simulink model "M10B39_es_V1"  (R2024b)
settings: Solver=ode23tb  StartTime=0.0  StopTime=20  FixedStep=0.001  RelTol=1e-3  EnableMultiTasking=on
InitFcn:
  | initAll;
values from neighbouring files (symbols this model uses):
  acom = 100    [initAll_V1.m]    (also in initAll_V2.m; initAll_V3.m; parameterinit.mat)
  AVm0 = [4.26082678503 4.656135219]    [parameterinit.mat]
  bcom = 50    [initAll_V1.m]    (also in initAll_V2.m; initAll_V3.m; parameterinit.mat)
  commun = 0*commun    [initAll_V1.m]    (also in initAll_V2.m; initAll_V3.m; parameterinit.mat = [0  0  0; 0  0  0; 0  0  0; 0  0  0])
  DataDelay = 0.0*DataDelay    [initAll_V1.m]    (also in initAll_V2.m; initAll_V3.m; parameterinit.mat = [0  0  0; 0  0  0; 0  0  0; 0  0  0])
  ESinit =     [parameterinit.mat]
  fB = 50    [initAll.m]    (also in initAll_V1.m; initAll_V2.m; initAll_V3.m; parameterinit.mat)
  Geninit = Generator_init(opdata,SynMach_in_gidx)    [initAll.m]    (also in initAll_V1.m; initAll_V2.m; initAll_V3.m = Generator_init(opdata_all,SynMach_in_gidx1); parameterinit.mat = )
  lam = 100    [initAll_V1.m]    (also in initAll_V2.m; initAll_V3.m; parameterinit.mat)
  SgridB = 100    [initAll.m]    (also in initAll_V1.m; initAll_V2.m; initAll_V3.m; parameterinit.mat)
  wB = 2*pi*fB    (= 314.159265359)    [initAll.m]    (also in initAll_V1.m; initAll_V2.m; initAll_V3.m; parameterinit.mat)
  Windinit =     [parameterinit.mat]
  YY_load = [3.65450097002 -2.05705688056 0 0 0 0 0 0 0 0 0 0 ... (1521 elements, 39x39)]    [parameterinit.mat]    (also in powerflowcaculate.m = full(YY))
undefined symbols (not defined in the file or in its folder): c1, c2, c3, c4, c5, c6, cp_nom, lambda_nom, P_wind_base, Pelec_base, Pnom
libraries: spsBistableLib x12, simulink_extras x4, slpidlib x1, simulink x1
(part 2 of 7)

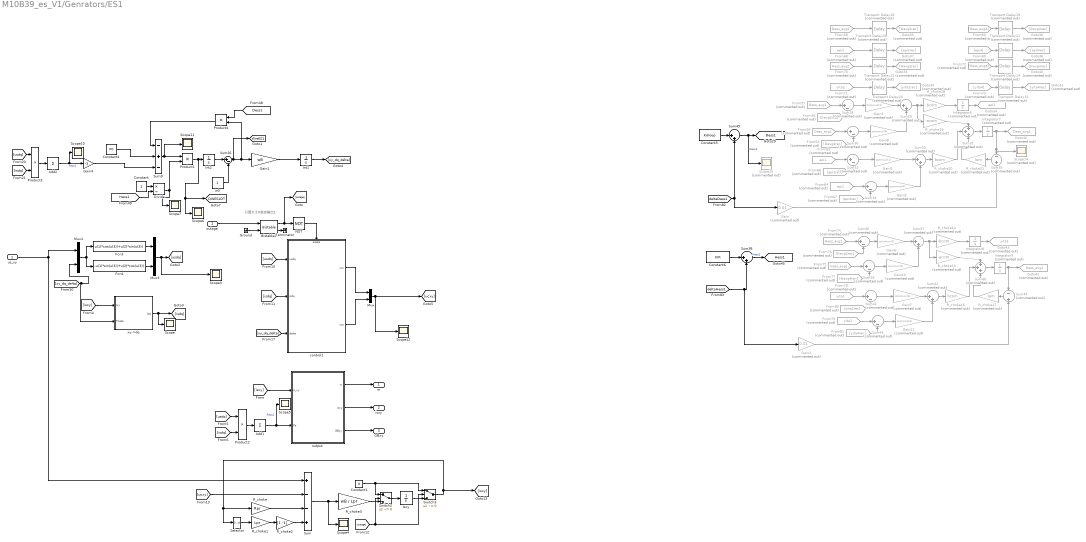
== system M10B39_es_V1/Genrators/ES1 ==
  note: 只要大于0就会输出1
  us_xy : Inport
  outage : Inport  Port=2
  " control1" : Subsystem
  Add1 : Sum  Inputs=+
  Add2 : Sum  Inputs=+
  Bistable2 : spsBistableLib/Bistable  Qpriority=Set  ic=0  Ts=0
      settings: LibrarySourceBlock=sps_lib/Control/Bistable
  Constant : Constant
  Constant1 : Constant  Value=0
  Constant4 : Constant  Value=P0
  Constant5 : Constant  Value=Kdroop
  Constant6 : Constant  Value=KIR
  Divide : Product  Inputs=*/
  Fcn3 : Fcn  Expr=u(1)*cos(u(3))+u(2)*sin(u(3))
  Fcn4 : Fcn  Expr=-u(1)*sin(u(3))+u(2)*cos(u(3))
  From57 : From  Commented=on  GotoTag=Dess_avg1  TagVisibility=global
  From58 : From  Commented=on  GotoTag=Dess_avg2  TagVisibility=global
  From59 : From  Commented=on  GotoTag=Dess_avg1  TagVisibility=global
  From60 : From  Commented=on  GotoTag=Dess_avg4  TagVisibility=global
  From61 : From  Commented=on  GotoTag=Davg2rec
  From62 : From  Commented=on  GotoTag=Davg4rec
  From63 : From  Commented=on  GotoTag=epi1  TagVisibility=global
  From64 : From  Commented=on  GotoTag=epi1  TagVisibility=global
  From66 : From  Commented=on  GotoTag=epi2rec
  From67 : From  Commented=on  GotoTag=epi4rec
  From68 : From  Commented=on  GotoTag=epi2  TagVisibility=global
  From69 : From  Commented=on  GotoTag=epi4  TagVisibility=global
  From70 : From  Commented=on  GotoTag=Hess_avg2  TagVisibility=global
  From71 : From  Commented=on  GotoTag=yita2  TagVisibility=global
  From72 : From  Commented=on  GotoTag=Hess_avg4  TagVisibility=global
  From73 : From  Commented=on  GotoTag=yita4  TagVisibility=global
  From74 : From  Commented=on  GotoTag=Hess_avg1  TagVisibility=global
  From75 : From  Commented=on  GotoTag=Hess_avg1  TagVisibility=global
  From76 : From  Commented=on  GotoTag=Havg2rec
  From77 : From  Commented=on  GotoTag=Havg4rec
  From78 : From  Commented=on  GotoTag=yita1  TagVisibility=global
  From79 : From  Commented=on  GotoTag=yita1  TagVisibility=global
  From80 : From  Commented=on  GotoTag=yita2rec
  From81 : From  Commented=on  GotoTag=yita4rec
  Gain : Gain  Commented=on  Gain=0.01
  Gain1 : Gain  Gain=wB  SaturateOnIntegerOverflow=on  OutDataTypeStr=Inherit: Same as input  ParamDataTypeStr=Inherit: Same as input
  Gain{8..11} (4 alike) : Gain  Commented=on  Gain=commun(4)
  Gain2 : Gain  Commented=on  Gain=0.01
  Gain{3,5..7} (4 alike) : Gain  Commented=on  Gain=commun(1)
  Gain4 : Gain  Gain=-1
  Goto32 : Goto  Commented=on  GotoTag=Dess_avg1  TagVisibility=global
  Goto33 : Goto  Commented=on  GotoTag=Havg2rec
  Goto34 : Goto  Commented=on  GotoTag=epi1  TagVisibility=global
  Goto35 : Goto  Commented=on  GotoTag=Davg2rec
  Goto36 : Goto  Commented=on  GotoTag=Davg4rec
  Goto37 : Goto  Commented=on  GotoTag=epi2rec
  Goto38 : Goto  Commented=on  GotoTag=epi4rec
  Goto39 : Goto  Commented=on  GotoTag=yita2rec
  Goto40 : Goto  Commented=on  GotoTag=Havg4rec
  Goto41 : Goto  Commented=on  GotoTag=yita4rec
  Goto42 : Goto  Commented=on  GotoTag=Hess_avg1  TagVisibility=global
  Goto43 : Goto  Commented=on  GotoTag=yita1  TagVisibility=global
  Ground : Ground
  Int1 : Integrator  InitialCondition=Dels_hvdc
  Int2 : Integrator  InitialCondition=1
  Integrator{6..9} (4 alike) : Integrator  Commented=on
  Isxy : Integrator  InitialCondition=[Is_xA_0 Is_yA_0]
  Mux : Mux  Inputs=2
  Mux3 : Mux  Inputs=2
  Mux4 : Mux  Inputs=2
  NOT : Logic  Operator=NOT  AllPortsSameDT=off  OutDataTypeStr=boolean
  Product1 : Product
  Product2 : Product  RndMeth=Zero
  Product3 : Product  RndMeth=Zero
  Product4 : Product
  R_choke : Gain  Gain=Rpr  SaturateOnIntegerOverflow=on  OutDataTypeStr=Inherit: Same as input  ParamDataTypeStr=Inherit: Same as input
  R_choke1 : Gain  Gain=Lpr  SaturateOnIntegerOverflow=on  OutDataTypeStr=Inherit: Same as input  ParamDataTypeStr=Inherit: Same as input
  R_choke14 : Gain  Commented=on  Gain=-bcom  SaturateOnIntegerOverflow=on  OutDataTypeStr=Inherit: Same as input  ParamDataTypeStr=Inherit: Same as input
  R_choke15 : Gain  Commented=on  Gain=-acom  SaturateOnIntegerOverflow=on  OutDataTypeStr=Inherit: Same as input  ParamDataTypeStr=Inherit: Same as input
  R_choke16 : Gain  Commented=on  Gain=bcom  SaturateOnIntegerOverflow=on  OutDataTypeStr=Inherit: Same as input  ParamDataTypeStr=Inherit: Same as input
  R_choke17 : Gain  Commented=on  Gain=lam  SaturateOnIntegerOverflow=on  OutDataTypeStr=Inherit: Same as input  ParamDataTypeStr=Inherit: Same as input
  R_choke18 : Gain  Commented=on  Gain=-bcom  SaturateOnIntegerOverflow=on  OutDataTypeStr=Inherit: Same as input  ParamDataTypeStr=Inherit: Same as input
  R_choke19 : Gain  Commented=on  Gain=-acom  SaturateOnIntegerOverflow=on  OutDataTypeStr=Inherit: Same as input  ParamDataTypeStr=Inherit: Same as input
  R_choke2 : Gain  Gain=[1 -1]  SaturateOnIntegerOverflow=on  OutDataTypeStr=Inherit: Same as input  ParamDataTypeStr=Inherit: Same as input
  R_choke20 : Gain  Commented=on  Gain=bcom  SaturateOnIntegerOverflow=on  OutDataTypeStr=Inherit: Same as input  ParamDataTypeStr=Inherit: Same as input
  R_choke21 : Gain  Commented=on  Gain=lam  SaturateOnIntegerOverflow=on  OutDataTypeStr=Inherit: Same as input  ParamDataTypeStr=Inherit: Same as input
  R_choke3 : Gain  Gain=wB / Lpr  SaturateOnIntegerOverflow=on  OutDataTypeStr=Inherit: Same as input  ParamDataTypeStr=Inherit: Same as input
  Scope{,3..7,10..12} (9 alike) : Scope
  Scope14 : Scope  Commented=on
  Scope15 : Scope  Commented=on
  Selector : Selector  InputPortWidth=2  IndexOptions=Index vector (dialog)  Indices=[2 1]  OutputSizes=1
  Sum : Sum  Inputs=+--+  SaturateOnIntegerOverflow=on
  Sum26 : Sum  Inputs=|+-  SaturateOnIntegerOverflow=on
  Sum{28,30,32,34,36,39,41,43} (8 alike) : Sum  Commented=on  Inputs=|+-  SaturateOnIntegerOverflow=on
  Sum{29,33,37,42} (4 alike) : Sum  Commented=on  Inputs=|++  SaturateOnIntegerOverflow=on
  Sum31 : Sum  Commented=on  Inputs=+++  SaturateOnIntegerOverflow=on
  Sum35 : Sum  Commented=on  Inputs=-+  SaturateOnIntegerOverflow=on
  Sum38 : Sum  Inputs=|++  SaturateOnIntegerOverflow=on
  Sum40 : Sum  Commented=on  Inputs=+++  SaturateOnIntegerOverflow=on
  Sum44 : Sum  Commented=on  Inputs=-+  SaturateOnIntegerOverflow=on
  Sum45 : Sum  Inputs=|++  SaturateOnIntegerOverflow=on
  Sum9 : Sum  Inputs=-+-  SaturateOnIntegerOverflow=on
  Switch2 : Switch  Criteria=u2 ~= 0  Threshold=0.5  InputSameDT=off
  Switch3 : Switch  Criteria=u2 ~= 0  Threshold=0.5  InputSameDT=off
  Terminator : Terminator
  Transport Delay{14..15,19,21} (4 alike) : TransportDelay  Commented=on  DelayTime=DataDelay(4,2)
  Transport Delay{18,20,22..23} (4 alike) : TransportDelay  Commented=on  DelayTime=DataDelay(2,1)
  output : Subsystem
  w0 : Constant
  xy->dq : Subsystem
  m : Outport
  isxy : Outport  Port=2
  GBxy : Outport  Port=3
  tag scope: DWES1DT=global, Dess1=global, Hess1=global, WreES1=global
  wires:
  Selector/1 -> R_choke1/1
  Sum/1 -> Scope4/1, R_choke3/1
  R_choke3/1 -> Switch2/3
  Ground/1 -> Bistable2/2
  R_choke2/1 -> Sum/4
  R_choke/1 -> Sum/3
  [ucxy] -> Sum/2
  output/1(m) -> m/1
  NOT/1 -> " control1"/Enable
  R_choke1/1 -> R_choke2/1
  Bistable2/1 -> NOT/1, [outage]
  Isxy/1 -> Switch3/3
  [isxy] -> xy->dq/1(Ixy)
  [isxy] -> output/1(is_xy)
  output/2(isxy) -> isxy/1
  [xy_dq_delta] -> " control1"/3(delta)
  xy->dq/1(Idq) -> [isdq], Scope/1
  Bistable2/2 -> Terminator/1
  outage/1 -> Bistable2/1
  [outage] -> Switch2/2, Switch3/2
  [isdq] -> " control1"/2(isdq)
  " control1"/1(ucx) -> Mux/1
  Switch2/1 -> Isxy/1
  Switch3/1 -> R_choke/1, Selector/1, [isxy]
  Mux/1 -> Scope12/1, [ucxy]
  [usdq] -> " control1"/1(usdq)
  output/3(GBxy) -> GBxy/1
  Constant1/1 -> Switch2/1, Switch3/1
  " control1"/2(ucy) -> Mux/2
  [usdq] -> Product2/1
  Add1/1 -> Scope5/1, output/2(Pe)  "Pess1"
  Product2/1 -> Add1/1
  [isdq] -> Product2/2
  Product1/1 -> Scope6/1, [DWES1DT], Int2/1
  Sum26/1 -> [WreES1], Product4/2, Gain1/1
  Int2/1 -> Sum26/1
  w0/1 -> Sum26/2
  Sum9/1 -> Product1/1, Scope11/1
  Constant/1 -> Divide/1
  Divide/1 -> Product1/2, Scope7/1
  [Hess1] -> Divide/2
  us_xy/1 -> Mux4/1, Sum/1
  Fcn3/1 -> Mux3/1
  Fcn4/1 -> Mux3/2
  Mux4/1 -> Fcn3/1, Fcn4/1
  [xy_dq_delta] -> Mux4/2, xy->dq/2(Theta)
  Mux3/1 -> Scope3/1, [usdq]
  Gain4/1 -> Sum9/3
  Constant4/1 -> Sum9/2
  Product4/1 -> Sum9/1
  Int1/1 -> [xy_dq_delta]
  Add2/1 -> Gain4/1, Scope10/1  "Pess1"
  [usdq] -> Product3/1
  [isdq] -> Product3/2
  Product3/1 -> Add2/1
  Transport Delay19/1 -> Goto36/1
  R_choke20/1 -> Sum31/2
  R_choke19/1 -> Sum31/1
  From57/1 -> Sum28/1
  From59/1 -> Sum30/1
  Sum38/1 -> [Hess1]  "Hess1"
  Sum45/1 -> Scope15/1, [Dess1]  "Dess1"
  Constant6/1 -> Sum38/1
  From64/1 -> Sum34/1
  R_choke21/1 -> Sum31/3
  Integrator6/1 -> Goto34/1
  Sum35/1 -> R_choke21/1
  Sum31/1 -> Integrator7/1
  Integrator7/1 -> Goto32/1, Scope14/1, Sum35/1
  Transport Delay21/1 -> Goto38/1
  From68/1 -> Transport Delay20/1
  From67/1 -> Sum34/2
  From62/1 -> Sum30/2
  From80/1 -> Sum41/2
  From78/1 -> Sum41/1
  Sum40/1 -> Integrator9/1
  [deltaDess1] -> Sum45/2, Gain/1
  R_choke18/1 -> Integrator6/1
  From77/1 -> Sum39/2
  From63/1 -> Sum32/1
  From76/1 -> Sum36/2
  Sum42/1 -> R_choke16/1
  From58/1 -> Transport Delay18/1
  Transport Delay20/1 -> Goto37/1
  Transport Delay14/1 -> Goto40/1
  From75/1 -> Sum39/1
  Integrator9/1 -> Goto42/1, Sum44/1
  Sum29/1 -> R_choke19/1, R_choke18/1
  From61/1 -> Sum28/2
  From71/1 -> Transport Delay23/1
  Sum37/1 -> R_choke15/1, R_choke14/1
  R_choke14/1 -> Integrator8/1
  Integrator8/1 -> Goto43/1
  Transport Delay18/1 -> Goto35/1
  R_choke17/1 -> Sum40/3
  R_choke15/1 -> Sum40/1
  R_choke16/1 -> Sum40/2
  From74/1 -> Sum36/1
  [deltaHess1] -> Sum38/2, Gain2/1
  Sum44/1 -> R_choke17/1
  Sum33/1 -> R_choke20/1
  Transport Delay23/1 -> Goto39/1
  From66/1 -> Sum32/2
  Transport Delay22/1 -> Goto33/1
  Transport Delay15/1 -> Goto41/1
  From70/1 -> Transport Delay22/1
  [Dess1] -> Product4/1
  Gain1/1 -> Int1/1
  From81/1 -> Sum43/2
  From79/1 -> Sum43/1
  Gain/1 -> Sum35/2
  Gain2/1 -> Sum44/2
  From60/1 -> Transport Delay19/1
  From69/1 -> Transport Delay21/1
  From72/1 -> Transport Delay14/1
  From73/1 -> Transport Delay15/1
  Gain3/1 -> Sum29/1
  Sum28/1 -> Gain3/1
  Gain5/1 -> Sum33/1
  Sum32/1 -> Gain5/1
  Sum36/1 -> Gain6/1
  Gain6/1 -> Sum37/1
  Gain7/1 -> Sum42/1
  Sum41/1 -> Gain7/1
  Sum30/1 -> Gain8/1
  Gain8/1 -> Sum29/2
  Sum34/1 -> Gain9/1
  Gain9/1 -> Sum33/2
  Sum39/1 -> Gain10/1
  Gain10/1 -> Sum37/2
  Sum43/1 -> Gain11/1
  Gain11/1 -> Sum42/2
  Constant5/1 -> Sum45/1

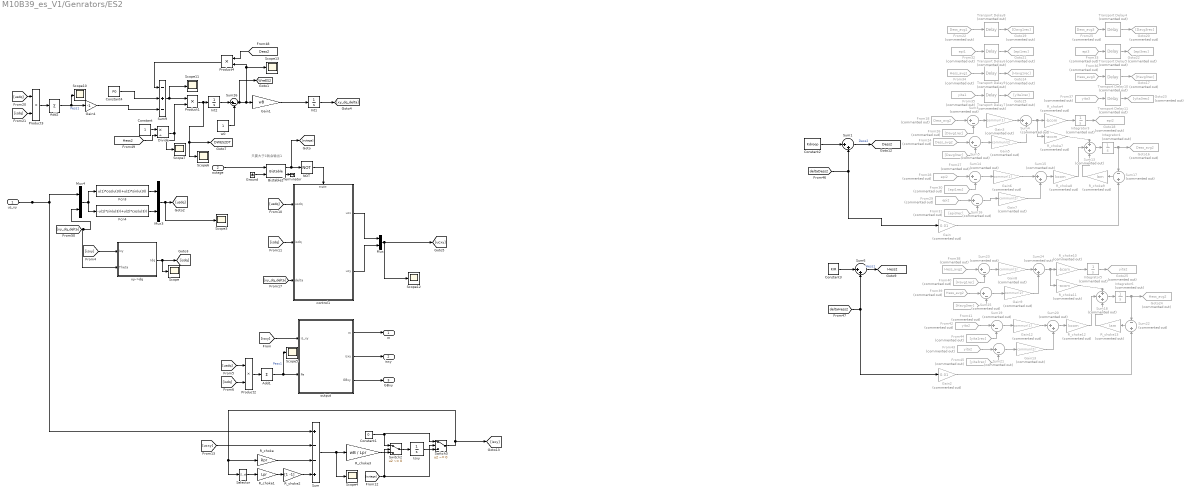
== system M10B39_es_V1/Genrators/ES2 ==
  note: 只要大于0就会输出1
  us_xy : Inport
  outage : Inport  Port=2
  " control1" : Subsystem
  Add1 : Sum  Inputs=+
  Add2 : Sum  Inputs=+
  Bistable2 : spsBistableLib/Bistable  Qpriority=Set  ic=0  Ts=0
      settings: LibrarySourceBlock=sps_lib/Control/Bistable
  Constant : Constant
  Constant1 : Constant  Value=0
  Constant2 : Constant  Value=Kdroop
  Constant3 : Constant  Value=KIR
  Constant4 : Constant  Value=P0
  Divide : Product  Inputs=*/
  Fcn3 : Fcn  Expr=u(1)*cos(u(3))+u(2)*sin(u(3))
  Fcn4 : Fcn  Expr=-u(1)*sin(u(3))+u(2)*cos(u(3))
  From18 : From  Commented=on  GotoTag=Dess_avg2  TagVisibility=global
  From22 : From  Commented=on  GotoTag=Dess_avg1  TagVisibility=global
  From24 : From  Commented=on  GotoTag=Dess_avg2  TagVisibility=global
  From25 : From  Commented=on  GotoTag=Dess_avg3  TagVisibility=global
  From26 : From  Commented=on  GotoTag=Davg1rec
  From27 : From  Commented=on  GotoTag=Davg3rec
  From28 : From  Commented=on  GotoTag=epi2  TagVisibility=global
  From29 : From  Commented=on  GotoTag=epi2  TagVisibility=global
  From30 : From  Commented=on  GotoTag=epi1rec
  From31 : From  Commented=on  GotoTag=epi3rec
  From32 : From  Commented=on  GotoTag=epi1  TagVisibility=global
  From33 : From  Commented=on  GotoTag=epi3  TagVisibility=global
  From34 : From  Commented=on  GotoTag=Hess_avg1  TagVisibility=global
  From35 : From  Commented=on  GotoTag=yita1  TagVisibility=global
  From36 : From  Commented=on  GotoTag=Hess_avg3  TagVisibility=global
  From37 : From  Commented=on  GotoTag=yita3  TagVisibility=global
  From38 : From  Commented=on  GotoTag=Hess_avg2  TagVisibility=global
  From39 : From  Commented=on  GotoTag=Hess_avg2  TagVisibility=global
  From40 : From  Commented=on  GotoTag=Havg1rec
  From41 : From  Commented=on  GotoTag=Havg3rec
  From42 : From  Commented=on  GotoTag=yita2  TagVisibility=global
  From43 : From  Commented=on  GotoTag=yita2  TagVisibility=global
  From44 : From  Commented=on  GotoTag=yita1rec
  From45 : From  Commented=on  GotoTag=yita3rec
  Gain : Gain  Commented=on  Gain=0.01
  Gain1 : Gain  Gain=wB  SaturateOnIntegerOverflow=on  OutDataTypeStr=Inherit: Same as input  ParamDataTypeStr=Inherit: Same as input
  Gain{3,6,8,12} (4 alike) : Gain  Commented=on  Gain=commun(1)
  Gain{5,7,9,13} (4 alike) : Gain  Commented=on  Gain=commun(2)
  Gain2 : Gain  Commented=on  Gain=0.01
  Gain4 : Gain  Gain=-1
  Goto14 : Goto  Commented=on  GotoTag=Havg1rec
  Goto15 : Goto  Commented=on  GotoTag=yita1rec
  Goto16 : Goto  Commented=on  GotoTag=Dess_avg2  TagVisibility=global
  Goto17 : Goto  Commented=on  GotoTag=Havg3rec
  Goto18 : Goto  Commented=on  GotoTag=epi2  TagVisibility=global
  Goto19 : Goto  Commented=on  GotoTag=Davg1rec
  Goto20 : Goto  Commented=on  GotoTag=Davg3rec
  Goto21 : Goto  Commented=on  GotoTag=epi1rec
  Goto22 : Goto  Commented=on  GotoTag=epi3rec
  Goto23 : Goto  Commented=on  GotoTag=yita3rec
  Goto24 : Goto  Commented=on  GotoTag=Hess_avg2  TagVisibility=global
  Goto25 : Goto  Commented=on  GotoTag=yita2  TagVisibility=global
  Ground : Ground
  Int1 : Integrator  InitialCondition=Dels_hvdc
  Int2 : Integrator  InitialCondition=1
  Integrator{3..6} (4 alike) : Integrator  Commented=on
  Isxy : Integrator  InitialCondition=[Is_xA_0 Is_yA_0]
  Mux : Mux  Inputs=2
  Mux3 : Mux  Inputs=2
  Mux4 : Mux  Inputs=2
  NOT : Logic  Operator=NOT  AllPortsSameDT=off  OutDataTypeStr=boolean
  Product1 : Product
  Product2 : Product  RndMeth=Zero
  Product3 : Product  RndMeth=Zero
  Product4 : Product
  R_choke : Gain  Gain=Rpr  SaturateOnIntegerOverflow=on  OutDataTypeStr=Inherit: Same as input  ParamDataTypeStr=Inherit: Same as input
  R_choke1 : Gain  Gain=Lpr  SaturateOnIntegerOverflow=on  OutDataTypeStr=Inherit: Same as input  ParamDataTypeStr=Inherit: Same as input
  R_choke10 : Gain  Commented=on  Gain=-bcom  SaturateOnIntegerOverflow=on  OutDataTypeStr=Inherit: Same as input  ParamDataTypeStr=Inherit: Same as input
  R_choke11 : Gain  Commented=on  Gain=-acom  SaturateOnIntegerOverflow=on  OutDataTypeStr=Inherit: Same as input  ParamDataTypeStr=Inherit: Same as input
  R_choke12 : Gain  Commented=on  Gain=bcom  SaturateOnIntegerOverflow=on  OutDataTypeStr=Inherit: Same as input  ParamDataTypeStr=Inherit: Same as input
  R_choke13 : Gain  Commented=on  Gain=lam  SaturateOnIntegerOverflow=on  OutDataTypeStr=Inherit: Same as input  ParamDataTypeStr=Inherit: Same as input
  R_choke2 : Gain  Gain=[1 -1]  SaturateOnIntegerOverflow=on  OutDataTypeStr=Inherit: Same as input  ParamDataTypeStr=Inherit: Same as input
  R_choke3 : Gain  Gain=wB / Lpr  SaturateOnIntegerOverflow=on  OutDataTypeStr=Inherit: Same as input  ParamDataTypeStr=Inherit: Same as input
  R_choke4 : Gain  Commented=on  Gain=-bcom  SaturateOnIntegerOverflow=on  OutDataTypeStr=Inherit: Same as input  ParamDataTypeStr=Inherit: Same as input
  R_choke7 : Gain  Commented=on  Gain=-acom  SaturateOnIntegerOverflow=on  OutDataTypeStr=Inherit: Same as input  ParamDataTypeStr=Inherit: Same as input
  R_choke8 : Gain  Commented=on  Gain=bcom  SaturateOnIntegerOverflow=on  OutDataTypeStr=Inherit: Same as input  ParamDataTypeStr=Inherit: Same as input
  R_choke9 : Gain  Commented=on  Gain=lam  SaturateOnIntegerOverflow=on  OutDataTypeStr=Inherit: Same as input  ParamDataTypeStr=Inherit: Same as input
  Scope{,3..7,10..13} (10 alike) : Scope
  Selector : Selector  InputPortWidth=2  IndexOptions=Index vector (dialog)  Indices=[2 1]  OutputSizes=1
  Sum : Sum  Inputs=+--+  SaturateOnIntegerOverflow=on
  Sum1 : Sum  Inputs=|++  SaturateOnIntegerOverflow=on
  Sum13 : Sum  Commented=on  Inputs=+++  SaturateOnIntegerOverflow=on
  Sum{3,5,14,16,19,21,23,25} (8 alike) : Sum  Commented=on  Inputs=|+-  SaturateOnIntegerOverflow=on
  Sum{4,15,20,24} (4 alike) : Sum  Commented=on  Inputs=|++  SaturateOnIntegerOverflow=on
  Sum17 : Sum  Commented=on  Inputs=-+  SaturateOnIntegerOverflow=on
  Sum18 : Sum  Commented=on  Inputs=+++  SaturateOnIntegerOverflow=on
  Sum22 : Sum  Commented=on  Inputs=-+  SaturateOnIntegerOverflow=on
  Sum26 : Sum  Inputs=|+-  SaturateOnIntegerOverflow=on
  Sum6 : Sum  Inputs=|++  SaturateOnIntegerOverflow=on
  Sum9 : Sum  Inputs=-+-  SaturateOnIntegerOverflow=on
  Switch2 : Switch  Criteria=u2 ~= 0  Threshold=0.5  InputSameDT=off
  Switch3 : Switch  Criteria=u2 ~= 0  Threshold=0.5  InputSameDT=off
  Terminator : Terminator
  Transport Delay{4..5,10..11} (4 alike) : TransportDelay  Commented=on  DelayTime=DataDelay(3,1)
  Transport Delay{6..9} (4 alike) : TransportDelay  Commented=on  DelayTime=DataDelay(1,2)
  output : Subsystem
  w0 : Constant
  xy->dq : Subsystem
  m : Outport
  isxy : Outport  Port=2
  GBxy : Outport  Port=3
  tag scope: DWES2DT=global, Dess2=global, Hess2=global, WreES2=global
  wires:
  Selector/1 -> R_choke1/1
  Sum/1 -> Scope4/1, R_choke3/1
  R_choke3/1 -> Switch2/3
  Ground/1 -> Bistable2/2
  R_choke2/1 -> Sum/4
  R_choke/1 -> Sum/3
  [ucxy] -> Sum/2
  output/1(m) -> m/1
  NOT/1 -> " control1"/Enable
  R_choke1/1 -> R_choke2/1
  Bistable2/1 -> NOT/1, [outage]
  Isxy/1 -> Switch3/3
  [isxy] -> xy->dq/1(Ixy)
  [isxy] -> output/1(is_xy)
  output/2(isxy) -> isxy/1
  [xy_dq_delta] -> " control1"/3(delta)
  xy->dq/1(Idq) -> [isdq], Scope/1
  Bistable2/2 -> Terminator/1
  outage/1 -> Bistable2/1
  [outage] -> Switch2/2, Switch3/2
  [isdq] -> " control1"/2(isdq)
  " control1"/1(ucx) -> Mux/1
  Switch2/1 -> Isxy/1
  Switch3/1 -> R_choke/1, Selector/1, [isxy]
  Mux/1 -> Scope12/1, [ucxy]
  [usdq] -> " control1"/1(usdq)
  output/3(GBxy) -> GBxy/1
  Constant1/1 -> Switch2/1, Switch3/1
  " control1"/2(ucy) -> Mux/2
  [usdq] -> Product2/1
  Add1/1 -> output/2(Pe), Scope5/1  "Pess1"
  Product2/1 -> Add1/1
  [isdq] -> Product2/2
  Product1/1 -> Scope6/1, [DWES2DT], Int2/1
  Sum26/1 -> [WreES2], Scope13/1, Product4/2, Gain1/1
  Int2/1 -> Sum26/1
  w0/1 -> Sum26/2
  Sum9/1 -> Product1/1, Scope11/1
  Constant/1 -> Divide/1
  Divide/1 -> Product1/2, Scope7/1
  [Hess2] -> Divide/2
  us_xy/1 -> Mux4/1, Sum/1
  Fcn3/1 -> Mux3/1
  Fcn4/1 -> Mux3/2
  Mux4/1 -> Fcn3/1, Fcn4/1
  [xy_dq_delta] -> Mux4/2, xy->dq/2(Theta)
  Mux3/1 -> Scope3/1, [usdq]
  Gain4/1 -> Sum9/3
  Constant4/1 -> Sum9/2
  Product4/1 -> Sum9/1
  Int1/1 -> [xy_dq_delta]
  Add2/1 -> Gain4/1, Scope10/1  "Pess1"
  [usdq] -> Product3/1
  [isdq] -> Product3/2
  Product3/1 -> Add2/1
  [Dess2] -> Product4/1
  Gain1/1 -> Int1/1
  From27/1 -> Sum5/2
  R_choke7/1 -> Sum13/1
  From44/1 -> Sum19/2
  R_choke8/1 -> Sum13/2
  From24/1 -> Sum5/1
  From18/1 -> Sum3/1
  Transport Delay9/1 -> Goto14/1
  From26/1 -> Sum3/2
  Transport Delay6/1 -> Goto21/1
  Integrator3/1 -> Goto18/1
  From30/1 -> Sum14/2
  Transport Delay5/1 -> Goto22/1
  Sum20/1 -> R_choke12/1
  Transport Delay4/1 -> Goto20/1
  From43/1 -> Sum21/1
  Transport Delay7/1 -> Goto15/1
  Sum17/1 -> R_choke9/1
  [deltaDess2] -> Sum1/2, Gain/1
  From39/1 -> Sum25/1
  Sum13/1 -> Integrator4/1
  R_choke10/1 -> Integrator5/1
  Sum15/1 -> R_choke8/1
  R_choke9/1 -> Sum13/3
  Constant3/1 -> Sum6/1
  Integrator4/1 -> Goto16/1, Sum17/1
  From29/1 -> Sum16/1
  [deltaHess2] -> Sum6/2, Gain2/1
  Transport Delay10/1 -> Goto17/1
  From31/1 -> Sum16/2
  Sum24/1 -> R_choke11/1, R_choke10/1
  Sum6/1 -> [Hess2]  "Hess1"
  From42/1 -> Sum19/1
  From28/1 -> Sum14/1
  R_choke12/1 -> Sum18/2
  From38/1 -> Sum23/1
  R_choke11/1 -> Sum18/1
  R_choke4/1 -> Integrator3/1
  Sum4/1 -> R_choke7/1, R_choke4/1
  From45/1 -> Sum21/2
  From40/1 -> Sum23/2
  From41/1 -> Sum25/2
  Transport Delay11/1 -> Goto23/1
  Sum22/1 -> R_choke13/1
  Integrator6/1 -> Goto24/1, Sum22/1
  Sum18/1 -> Integrator6/1
  Integrator5/1 -> Goto25/1
  R_choke13/1 -> Sum18/3
  Transport Delay8/1 -> Goto19/1
  Sum1/1 -> [Dess2]  "Dess2"
  Constant2/1 -> Sum1/1
  Gain/1 -> Sum17/2
  Gain2/1 -> Sum22/2
  From22/1 -> Transport Delay8/1
  From32/1 -> Transport Delay6/1
  From34/1 -> Transport Delay9/1
  From35/1 -> Transport Delay7/1
  From25/1 -> Transport Delay4/1
  From33/1 -> Transport Delay5/1
  From36/1 -> Transport Delay10/1
  From37/1 -> Transport Delay11/1
  Gain3/1 -> Sum4/1
  Sum3/1 -> Gain3/1
  Sum5/1 -> Gain5/1
  Gain5/1 -> Sum4/2
  Gain6/1 -> Sum15/1
  Sum14/1 -> Gain6/1
  Sum16/1 -> Gain7/1
  Gain7/1 -> Sum15/2
  Sum23/1 -> Gain8/1
  Gain8/1 -> Sum24/1
  Sum25/1 -> Gain9/1
  Gain9/1 -> Sum24/2
  Gain12/1 -> Sum20/1
  Sum19/1 -> Gain12/1
  Sum21/1 -> Gain13/1
  Gain13/1 -> Sum20/2

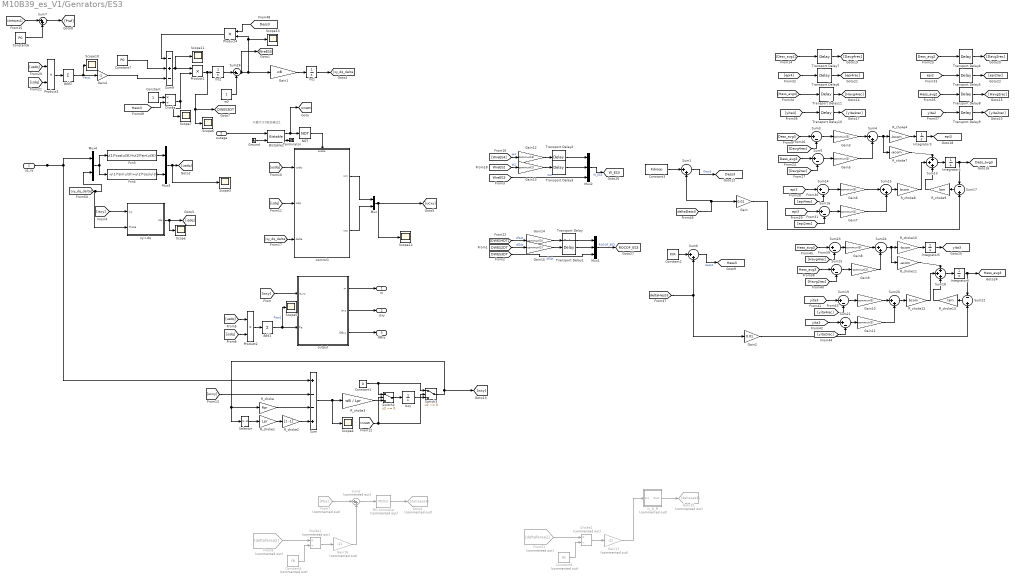
== system M10B39_es_V1/Genrators/ES3 ==
  note: 只要大于0就会输出1
  us_xy : Inport
  outage : Inport  Port=2
  " control1" : Subsystem
  Add1 : Sum  Inputs=+
  Add2 : Sum  Inputs=+
  Bistable2 : spsBistableLib/Bistable  Qpriority=Set  ic=0  Ts=0
  Constant : Constant
  Constant1 : Constant  Value=0
  Constant2 : Constant  Value=KIR
  Constant3 : Constant  Value=Kdroop
  Constant4 : Constant  Commented=on  Value=fB
  Constant5 : Constant  Commented=on  Value=fB
  Constant6 : Constant  Value=P0
  Constant7 : Constant  Value=P0
  Divide : Product  Inputs=*/
  Divide1 : Product  Commented=on  Inputs=*/
  Divide2 : Product  Commented=on  Inputs=*/
  Fcn3 : Fcn  Expr=u(1)*cos(u(3))+u(2)*sin(u(3))
  Fcn4 : Fcn  Expr=-u(1)*sin(u(3))+u(2)*cos(u(3))
  From51 : From  Commented=on  GotoTag=deltafarea2  TagVisibility=global
  From7 : From  Commented=on  GotoTag=Ptie  TagVisibility=global
  From8 : From  Commented=on  GotoTag=deltafarea2  TagVisibility=global
  Gain : Gain  Gain=0.01
  Gain1 : Gain  Gain=wB  SaturateOnIntegerOverflow=on  OutDataTypeStr=Inherit: Same as input  ParamDataTypeStr=Inherit: Same as input
  Gain{3,6,8,10,12,14} (6 alike) : Gain  Gain=commun(3)
  Gain{5,7,9,11,13,15} (6 alike) : Gain  Gain=commun(2)
  Gain16 : Gain  Commented=on  Gain=-21
  Gain17 : Gain  Commented=on  Gain=-21
  Gain2 : Gain  Gain=0.01
  Gain4 : Gain  Gain=-1
  Goto10 : Goto  Commented=on  GotoTag=deltapes3
  Goto6 : Goto  Commented=on  GotoTag=deltapes3
  Ground : Ground
  Int1 : Integrator  InitialCondition=Dels_hvdc
  Int2 : Integrator  InitialCondition=1
  Integrator{3..6} (4 alike) : Integrator
  Isxy : Integrator  InitialCondition=[Is_xA_0 Is_yA_0]
  Mux : Mux  Inputs=2
  Mux1 : Mux  Inputs=3
  Mux2 : Mux  Inputs=3
  Mux3 : Mux  Inputs=2
  Mux4 : Mux  Inputs=2
  NOT : Logic  Operator=NOT  AllPortsSameDT=off  OutDataTypeStr=boolean
  PID Controller : slpidlib/PID Controller  Commented=on  Controller=PID  Form=Parallel  TimeDomain=Continuous-time  UseExternalTs=off  SampleTime=-1  IntegratorMethod=Forward Euler  FilterMethod=Forward Euler  ControllerParametersSource=internal  P=1  I=1  UseKiTs=off  D=0  UseExternalDerivativeSource=off  N=100  UseFilter=on  TunerSelectOption=Transfer Function Based (PID Tuner App)  InitialConditionSource=internal  InitialConditionForIntegrator=0  InitialConditionForFilter=0  DifferentiatorICPrevScaledInput=0  ExternalReset=none  TrackingMode=off  Kt=1  LimitOutput=off  SatLimitsSource=internal  UpperSaturationLimit=inf  LowerSaturationLimit=-inf  LinearizeAsGain=on  AntiWindupMode=none  Kb=1  LimitIntegrator=off  UpperIntegratorSaturationLimit=inf  LowerIntegratorSaturationLimit=-inf  POutMin=[]  POutMax=[]  IOutMin=[]  IOutMax=[]  DOutMin=[]  DOutMax=[]  NOutMin=[]  NOutMax=[]  SumOutMin=[]  SumOutMax=[]  SaturationOutMin=[]  SaturationOutMax=[]  PParamMin=[]  PParamMax=[]  IParamMin=[]  IParamMax=[]  DParamMin=[]  DParamMax=[]  NParamMin=[]  NParamMax=[]  KbParamMin=[]  KbParamMax=[]  KtParamMin=[]  KtParamMax=[]  KbOutMin=[]  KbOutMax=[]  KtOutMin=[]  KtOutMax=[]  IntegratorOutMin=[]  IntegratorOutMax=[]  FilterOutMin=[]  FilterOutMax=[]  SumI1OutMin=[]  SumI1OutMax=[]  SumI2OutMin=[]  SumI2OutMax=[]  SumI3OutMin=[]  SumI3OutMax=[]  SumI4OutMin=[]  SumI4OutMax=[]  SumDOutMin=[]  SumDOutMax=[]  DifferentiatorOutMin=[]  DifferentiatorOutMax=[]  FilterDiffOutCoefMin=[]  FilterDiffOutCoefMax=[]  ReciprocalOutMin=[]  ReciprocalOutMax=[]  SumDenOutMin=[]  SumDenOutMax=[]  SumNumOutMin=[]  SumNumOutMax=[]  DivideOutMin=[]  DivideOutMax=[]  UdiffTsProdOutMin=[]  UdiffTsProdOutMax=[]  NTsProdOutMin=[]  NTsProdOutMax=[]  UintegralTsProdOutMin=[]  UintegralTsProdOutMax=[]  UngainTsProdOutMin=[]  UngainTsProdOutMax=[]  ClampingZeroOutDataTypeStr=Inherit: Inherit via back propagation  ClampingZeroOutMin=[]  ClampingZeroOutMax=[]  FilterDenConstantOutDataTypeStr=Inherit: Inherit via back propagation  FilterDenConstantOutMin=[]  FilterDenConstantOutMax=[]  PCopyOutDataTypeStr=Inherit: Inherit via back propagation  PCopyOutMin=[]  PCopyOutMax=[]  NCopyOutDataTypeStr=Inherit: Inherit via back propagation  NCopyOutMin=[]  NCopyOutMax=[]  IntegratorContinuousStateAttributes=''  IntegratorStateMustResolveToSignalObject=off  IntegratorRTWStateStorageClass=Auto  FilterContinuousStateAttributes=''  FilterStateMustResolveToSignalObject=off  FilterRTWStateStorageClass=Auto  ParallelPVariant=InternalParameters  IdealPVariant=Disabled  IVariant=InternalParameters  DVariant=InternalParameters  IntegratorVariant=Continuous  SatVariant=Disabled  AWVariant=Passthrough  PCopyVariant=Disabled  TRVariant=Disabled  FdbkBlocksVariant=Forward  IdealPFdbkVariant=Disabled  SatFdbkVariant=Disabled  DerivativeFilterVariant=ContFilter  NVariant=InternalParameters  NCopyVariant=Disabled  FilterICVariant=InternalICsFilter  IntegratorICVariant=InternalICs  ExternalResetVariant=Disabled  TRSumVariant=Passthrough  SumFdbkVariant=Disabled  SumVariant=Sum_PID  TsampFilterVariant=InternalTs  TsampNgainVariant=Passthrough  TsampIntegralVariant=Disabled_SignalSpec  ExternalSaturationOutDataTypeStr=Inherit: Same as second input  DerivativeSourceVariant=ErrorSignal  PreIntVariant=InternalPreInt
  Product1 : Product
  Product2 : Product  RndMeth=Zero
  Product3 : Product  RndMeth=Zero
  Product4 : Product
  R_choke : Gain  Gain=Rpr  SaturateOnIntegerOverflow=on  OutDataTypeStr=Inherit: Same as input  ParamDataTypeStr=Inherit: Same as input
  R_choke1 : Gain  Gain=Lpr  SaturateOnIntegerOverflow=on  OutDataTypeStr=Inherit: Same as input  ParamDataTypeStr=Inherit: Same as input
  R_choke10 : Gain  Gain=-bcom  SaturateOnIntegerOverflow=on  OutDataTypeStr=Inherit: Same as input  ParamDataTypeStr=Inherit: Same as input
  R_choke11 : Gain  Gain=-acom  SaturateOnIntegerOverflow=on  OutDataTypeStr=Inherit: Same as input  ParamDataTypeStr=Inherit: Same as input
  R_choke12 : Gain  Gain=bcom  SaturateOnIntegerOverflow=on  OutDataTypeStr=Inherit: Same as input  ParamDataTypeStr=Inherit: Same as input
  R_choke13 : Gain  Gain=lam  SaturateOnIntegerOverflow=on  OutDataTypeStr=Inherit: Same as input  ParamDataTypeStr=Inherit: Same as input
  R_choke2 : Gain  Gain=[1 -1]  SaturateOnIntegerOverflow=on  OutDataTypeStr=Inherit: Same as input  ParamDataTypeStr=Inherit: Same as input
  R_choke3 : Gain  Gain=wB / Lpr  SaturateOnIntegerOverflow=on  OutDataTypeStr=Inherit: Same as input  ParamDataTypeStr=Inherit: Same as input
  R_choke4 : Gain  Gain=-bcom  SaturateOnIntegerOverflow=on  OutDataTypeStr=Inherit: Same as input  ParamDataTypeStr=Inherit: Same as input
  R_choke7 : Gain  Gain=-acom  SaturateOnIntegerOverflow=on  OutDataTypeStr=Inherit: Same as input  ParamDataTypeStr=Inherit: Same as input
  R_choke8 : Gain  Gain=bcom  SaturateOnIntegerOverflow=on  OutDataTypeStr=Inherit: Same as input  ParamDataTypeStr=Inherit: Same as input
  R_choke9 : Gain  Gain=lam  SaturateOnIntegerOverflow=on  OutDataTypeStr=Inherit: Same as input  ParamDataTypeStr=Inherit: Same as input
  Scope{,3..7,10..13} (10 alike) : Scope
  Selector : Selector  InputPortWidth=2  IndexOptions=Index vector (dialog)  Indices=[2 1]  OutputSizes=1
  Sum : Sum  Inputs=+--+  SaturateOnIntegerOverflow=on
  Sum{1,4,6,15,20,24} (6 alike) : Sum  Inputs=|++  SaturateOnIntegerOverflow=on
  Sum13 : Sum  Inputs=+++  SaturateOnIntegerOverflow=on
  Sum{3,5,14,16,19,21,23,25..26} (9 alike) : Sum  Inputs=|+-  SaturateOnIntegerOverflow=on
  Sum17 : Sum  Inputs=-+  SaturateOnIntegerOverflow=on
  Sum18 : Sum  Inputs=+++  SaturateOnIntegerOverflow=on
  Sum2 : Sum  Commented=on  Inputs=|++
  Sum22 : Sum  Inputs=-+  SaturateOnIntegerOverflow=on
  Sum7 : Sum  Inputs=|++
  Sum9 : Sum  Inputs=-+-  SaturateOnIntegerOverflow=on
  Switch2 : Switch  Criteria=u2 ~= 0  Threshold=0.5  InputSameDT=off
  Switch3 : Switch  Criteria=u2 ~= 0  Threshold=0.5  InputSameDT=off
  Terminator : Terminator
  Transport Delay{,2,6..7,10..11} (6 alike) : TransportDelay  DelayTime=DataDelay(4,1)
  Transport Delay{1,3..5,8..9} (6 alike) : TransportDelay  DelayTime=DataDelay(2,2)
  in_D_PI : Subsystem  Commented=on  mask{KP_=0.1, KI_=0.1, Upper_limit=inf, Lower_limit=-inf, Upper_saturation_limit=inf, Lower_saturation_limit=-inf, integrator_init=Md_A_0}
      mask prompts: KP_ "比例系数P"; KI_ "积分系数I"; Upper_limit "限幅上限"; Lower_limit "限幅下限"; Upper_saturation_limit "积分饱和上限"; Lower_saturation_limit "积分饱和下限"; integrator_init "积分初始值"
      mask DialogControl Container4 Prompt: 控制参数
      mask DialogControl Container5 Prompt: 初始值
      mask Display: disp('PI')
  output : Subsystem
  w0 : Constant
  xy->dq : Subsystem
  m : Outport
  isxy : Outport  Port=2
  GBxy : Outport  Port=3
  tag scope: DWES3DT=global, Dess3=global, Dess_avg3=global, Hess3=global, Hess_avg3=global, ROCOF_ES3=global, W_ES3=global, WreES3=global, epi3=global, yita3=global
  wires:
  Selector/1 -> R_choke1/1
  Sum/1 -> Scope4/1, R_choke3/1
  R_choke3/1 -> Switch2/3
  Ground/1 -> Bistable2/2
  R_choke2/1 -> Sum/4
  R_choke/1 -> Sum/3
  [ucxy] -> Sum/2
  output/1(m) -> m/1
  NOT/1 -> " control1"/Enable
  R_choke1/1 -> R_choke2/1
  Bistable2/1 -> NOT/1, [outage]
  Isxy/1 -> Switch3/3
  [isxy] -> xy->dq/1(Ixy)
  [isxy] -> output/1(is_xy)
  output/2(isxy) -> isxy/1
  [xy_dq_delta] -> " control1"/3(delta)
  xy->dq/1(Idq) -> [isdq], Scope/1
  Bistable2/2 -> Terminator/1
  outage/1 -> Bistable2/1
  [outage] -> Switch2/2, Switch3/2
  [isdq] -> " control1"/2(isdq)
  " control1"/1(ucx) -> Mux/1
  Switch2/1 -> Isxy/1
  Switch3/1 -> R_choke/1, Selector/1, [isxy]
  Mux/1 -> Scope12/1, [ucxy]
  [usdq] -> " control1"/1(usdq)
  output/3(GBxy) -> GBxy/1
  Constant1/1 -> Switch2/1, Switch3/1
  " control1"/2(ucy) -> Mux/2
  [usdq] -> Product2/1
  Add1/1 -> Scope5/1, output/2(Pe)  "Pess1"
  Product2/1 -> Add1/1
  [isdq] -> Product2/2
  Product1/1 -> Scope6/1, [DWES3DT], Int2/1
  Int2/1 -> Sum26/1
  w0/1 -> Sum26/2
  Sum9/1 -> Product1/1, Scope11/1
  Constant/1 -> Divide/1
  Divide/1 -> Product1/2, Scope7/1
  [Hess3] -> Divide/2
  us_xy/1 -> Mux4/1, Sum/1
  Fcn3/1 -> Mux3/1
  Fcn4/1 -> Mux3/2
  Mux4/1 -> Fcn3/1, Fcn4/1
  [xy_dq_delta] -> Mux4/2, xy->dq/2(Theta)
  Mux3/1 -> Scope3/1, [usdq]
  Gain4/1 -> Sum9/3
  Product4/1 -> Sum9/1
  Int1/1 -> [xy_dq_delta]
  Add2/1 -> Gain4/1, Scope10/1  "Pess1"
  [usdq] -> Product3/1
  [isdq] -> Product3/2
  Product3/1 -> Add2/1
  [Dess3] -> Product4/1
  Gain1/1 -> Int1/1
  R_choke8/1 -> Sum13/2
  Transport Delay9/1 -> [yita2rec]
  Sum6/1 -> [Hess3]  "Hess3"
  [yita3] -> Sum21/1
  R_choke4/1 -> Integrator3/1
  [WreES3] -> Mux2/3  "W3"
  Transport Delay/1 -> Mux1/1
  [Havg4rec] -> Sum23/2
  [Dess_avg3] -> Sum3/1
  [Havg2rec] -> Sum25/2
  [Dess_avg3] -> Sum5/1
  [Davg2rec] -> Sum5/2
  [DWES3DT] -> Mux1/3  "df3dt"
  Transport Delay4/1 -> [Davg2rec]
  Mux2/1 -> [W_ES3]  "W_ES3"
  [Hess_avg3] -> Sum23/1
  Transport Delay1/1 -> Mux1/2
  Constant2/1 -> Sum6/1
  Sum1/1 -> [Dess3]  "Dess3"
  Constant3/1 -> Sum1/1
  [epi3] -> Sum14/1
  Sum20/1 -> R_choke12/1
  [Davg4rec] -> Sum3/2
  [epi4rec] -> Sum14/2
  [epi3] -> Sum16/1
  R_choke13/1 -> Sum18/3
  Sum24/1 -> R_choke11/1, R_choke10/1
  R_choke7/1 -> Sum13/1
  R_choke9/1 -> Sum13/3
  [yita2rec] -> Sum21/2
  Sum4/1 -> R_choke7/1, R_choke4/1
  R_choke11/1 -> Sum18/1
  Transport Delay5/1 -> [epi2rec]
  Transport Delay2/1 -> Mux2/1
  Integrator5/1 -> [yita3]
  Transport Delay3/1 -> Mux2/2
  Transport Delay10/1 -> [yita4rec]
  [Hess_avg3] -> Sum25/1
  Integrator6/1 -> [Hess_avg3], Sum22/1
  Transport Delay7/1 -> [Davg4rec]
  R_choke10/1 -> Integrator5/1
  Integrator3/1 -> [epi3]
  Transport Delay6/1 -> [epi4rec]
  Transport Delay11/1 -> [Havg4rec]
  Transport Delay8/1 -> [Havg2rec]
  Sum17/1 -> R_choke9/1
  [epi2rec] -> Sum16/2
  Sum22/1 -> R_choke13/1
  Sum15/1 -> R_choke8/1
  [yita4rec] -> Sum19/2
  R_choke12/1 -> Sum18/2
  Sum18/1 -> Integrator6/1
  [deltaDess3] -> Sum1/2, Gain/1
  Mux1/1 -> [ROCOF_ES3]  "ROCOF_ES3"
  Integrator4/1 -> [Dess_avg3], Sum17/1
  Sum13/1 -> Integrator4/1
  [yita3] -> Sum19/1
  Sum26/1 -> [WreES3], Gain1/1, Scope13/1, Product4/2
  Gain/1 -> Sum17/2
  Gain2/1 -> Sum22/2
  [Dess_avg4] -> Transport Delay7/1
  [epi4] -> Transport Delay6/1
  [Hess_avg4] -> Transport Delay11/1
  [yita4] -> Transport Delay10/1
  [yita2] -> Transport Delay9/1
  [Hess_avg2] -> Transport Delay8/1
  [epi2] -> Transport Delay5/1
  [Dess_avg2] -> Transport Delay4/1
  [WreES4] -> Gain12/1  "W4"
  Gain12/1 -> Transport Delay2/1
  [WreES2] -> Gain13/1  "W2"
  Gain13/1 -> Transport Delay3/1
  Gain14/1 -> Transport Delay/1
  [DWES4DT] -> Gain14/1  "df1dt"
  Gain15/1 -> Transport Delay1/1
  [DWES2DT] -> Gain15/1  "df2dt"
  [deltaHess3] -> Gain2/1, Sum6/2
  Gain3/1 -> Sum4/1
  Sum3/1 -> Gain3/1
  Sum5/1 -> Gain5/1
  Gain5/1 -> Sum4/2
  Sum14/1 -> Gain6/1
  Gain6/1 -> Sum15/1
  Sum16/1 -> Gain7/1
  Gain7/1 -> Sum15/2
  Sum23/1 -> Gain8/1
  Gain8/1 -> Sum24/1
  Gain9/1 -> Sum24/2
  Sum25/1 -> Gain9/1
  Sum19/1 -> Gain10/1
  Gain10/1 -> Sum20/1
  Gain11/1 -> Sum20/2
  Sum21/1 -> Gain11/1
  Divide1/1 -> Gain16/1
  Constant5/1 -> Divide1/2
  From7/1 -> Sum2/1
  From8/1 -> Divide1/1
  Gain16/1 -> Sum2/2
  Sum2/1 -> PID Controller/1
  PID Controller/1 -> Goto6/1
  [deltapes3] -> Sum7/1
  Constant6/1 -> Sum7/2
  Sum7/1 -> [Pref]
  Constant7/1 -> Sum9/2
  From51/1 -> Divide2/1
  Constant4/1 -> Divide2/2
  Divide2/1 -> Gain17/1
  in_D_PI/1(Out1) -> Goto10/1
  Gain17/1 -> in_D_PI/1(In1)

== system M10B39_es_V1/Genrators/Generator1 ==
  Vgxy : Inport
  Trip : Inport  Port=2
  Bistable2 : spsBistableLib/Bistable  Qpriority=Set  ic=0  Ts=0
      settings: LibrarySourceBlock=sps_lib/Control/Bistable
  Constant : Constant  Value=[0,0,0,0]
  Excitation System ST1A1 : Subsystem
  Governor : Subsystem
  Ground : Ground
  "Machine Equations " : Subsystem
  Mechanical DE : Subsystem
  Output : Subsystem
  PSS1 : Subsystem
  Scope{,1..3,5} (5 alike) : Scope
  Switch4 : Switch  Criteria=u2 ~= 0  Threshold=0.5  InputSameDT=off
  Terminator : Terminator
  pu->pu : Gain  Gain=SgenB./SgridB
  pu->pu1 : Gain  Gain=SgenB./SgridB
  m : Outport
  Igxy1 : Outport  Port=2
  GBxy : Outport  Port=3
  wires:
  pu->pu1/1 -> [GBxy]
  pu->pu/1 -> [Igxy1]
  "Machine Equations "/3(GBxy) -> Switch4/3
  Constant/1 -> Switch4/1
  Switch4/1 -> pu->pu1/1
  [Trip] -> Switch4/2
  [Trip] -> PSS1/2(Trip)
  [Trip] -> Governor/2(Trip)
  [Trip] -> Mechanical DE/3(Trip)
  [Trip] -> Excitation System ST1A1/2(Trip)
  [Trip] -> "Machine Equations "/4(Trip)
  Bistable2/2 -> Terminator/1
  Trip/1 -> Bistable2/1
  Ground/1 -> Bistable2/2
  Bistable2/1 -> [Trip]
  [Vg] -> Output/6(Vg)
  Output/1(m) -> m/1
  Output/3(GBxy) -> GBxy/1
  Output/2(Igxy1) -> Igxy1/1
  [Igxy1] -> Output/1(Igxy1in)
  [GBxy] -> Output/2(GBxyin)
  [delta] -> Output/3(deltain)
  [f] -> Output/5(fin)
  [Pe] -> Output/4(Pein)
  Mechanical DE/1(delta) -> "Machine Equations "/1(delta), [delta], Scope/1
  Governor/1(dPm) -> Scope3/1, Mechanical DE/2(dPm)
  PSS1/1(Upss) -> Scope2/1, Excitation System ST1A1/1(Upss)
  Mechanical DE/2(w) -> [f], PSS1/1(w), Governor/1(w)
  "Machine Equations "/2(Igxy1) -> pu->pu/1
  Vgxy/1 -> "Machine Equations "/2(Vgxy)
  "Machine Equations "/4(Vg) -> [Vg], Excitation System ST1A1/3(Vg)
  "Machine Equations "/1(Pe) -> [Pe], Mechanical DE/1(Pe), Scope1/1
  Excitation System ST1A1/1(Ef) -> "Machine Equations "/3(Ef), Scope5/1

== system M10B39_es_V1/Genrators/Generator2 ==
  Vgxy : Inport
  Trip : Inport  Port=2
  Bistable2 : spsBistableLib/Bistable  Qpriority=Set  ic=0  Ts=0
      settings: LibrarySourceBlock=sps_lib/Control/Bistable
  Constant : Constant  Value=[0,0,0,0]
  Excitation System ST1A1 : Subsystem
  Governor : Subsystem
  Ground : Ground
  "Machine Equations " : Subsystem
  Mechanical DE : Subsystem
  Output : Subsystem
  PSS1 : Subsystem
  Scope{,1..3,5} (5 alike) : Scope
  Switch4 : Switch  Criteria=u2 ~= 0  Threshold=0.5  InputSameDT=off
  Terminator : Terminator
  pu->pu : Gain  Gain=SgenB./SgridB
  pu->pu1 : Gain  Gain=SgenB./SgridB
  m : Outport
  Igxy1 : Outport  Port=2
  GBxy : Outport  Port=3
  wires:
  pu->pu1/1 -> [GBxy]
  pu->pu/1 -> [Igxy1]
  "Machine Equations "/3(GBxy) -> Switch4/3
  Constant/1 -> Switch4/1
  Switch4/1 -> pu->pu1/1
  [Trip] -> Switch4/2
  [Trip] -> PSS1/2(Trip)
  [Trip] -> Governor/2(Trip)
  [Trip] -> Mechanical DE/3(Trip)
  [Trip] -> Excitation System ST1A1/2(Trip)
  [Trip] -> "Machine Equations "/4(Trip)
  Bistable2/2 -> Terminator/1
  Trip/1 -> Bistable2/1
  Ground/1 -> Bistable2/2
  Bistable2/1 -> [Trip]
  [Vg] -> Output/6(Vg)
  Output/1(m) -> m/1
  Output/3(GBxy) -> GBxy/1
  Output/2(Igxy1) -> Igxy1/1
  [Igxy1] -> Output/1(Igxy1in)
  [GBxy] -> Output/2(GBxyin)
  [delta] -> Output/3(deltain)
  [f] -> Output/5(fin)
  [Pe] -> Output/4(Pein)
  Mechanical DE/1(delta) -> "Machine Equations "/1(delta), [delta], Scope/1
  Governor/1(dPm) -> Scope3/1, Mechanical DE/2(dPm)
  PSS1/1(Upss) -> Scope2/1, Excitation System ST1A1/1(Upss)
  Mechanical DE/2(w) -> [f], PSS1/1(w), Governor/1(w)
  "Machine Equations "/2(Igxy1) -> pu->pu/1
  Vgxy/1 -> "Machine Equations "/2(Vgxy)
  "Machine Equations "/4(Vg) -> [Vg], Excitation System ST1A1/3(Vg)
  "Machine Equations "/1(Pe) -> [Pe], Mechanical DE/1(Pe), Scope1/1
  Excitation System ST1A1/1(Ef) -> "Machine Equations "/3(Ef), Scope5/1

== system M10B39_es_V1/Genrators/Generator3 ==
  Vgxy : Inport
  Trip : Inport  Port=2
  Bistable2 : spsBistableLib/Bistable  Qpriority=Set  ic=0  Ts=0
      settings: LibrarySourceBlock=sps_lib/Control/Bistable
  Constant : Constant  Value=[0,0,0,0]
  Excitation System ST1A1 : Subsystem
  Governor : Subsystem
  Ground : Ground
  "Machine Equations " : Subsystem
  Mechanical DE : Subsystem
  Output : Subsystem
  PSS1 : Subsystem
  Scope{,1..3,5} (5 alike) : Scope
  Switch4 : Switch  Criteria=u2 ~= 0  Threshold=0.5  InputSameDT=off
  Terminator : Terminator
  pu->pu : Gain  Gain=SgenB./SgridB
  pu->pu1 : Gain  Gain=SgenB./SgridB
  m : Outport
  Igxy1 : Outport  Port=2
  GBxy : Outport  Port=3
  wires:
  pu->pu1/1 -> [GBxy]
  pu->pu/1 -> [Igxy1]
  "Machine Equations "/3(GBxy) -> Switch4/3
  Constant/1 -> Switch4/1
  Switch4/1 -> pu->pu1/1
  [Trip] -> Switch4/2
  [Trip] -> PSS1/2(Trip)
  [Trip] -> Governor/2(Trip)
  [Trip] -> Mechanical DE/3(Trip)
  [Trip] -> Excitation System ST1A1/2(Trip)
  [Trip] -> "Machine Equations "/4(Trip)
  Bistable2/2 -> Terminator/1
  Trip/1 -> Bistable2/1
  Ground/1 -> Bistable2/2
  Bistable2/1 -> [Trip]
  [Vg] -> Output/6(Vg)
  Output/1(m) -> m/1
  Output/3(GBxy) -> GBxy/1
  Output/2(Igxy1) -> Igxy1/1
  [Igxy1] -> Output/1(Igxy1in)
  [GBxy] -> Output/2(GBxyin)
  [delta] -> Output/3(deltain)
  [f] -> Output/5(fin)
  [Pe] -> Output/4(Pein)
  Mechanical DE/1(delta) -> "Machine Equations "/1(delta), [delta], Scope/1
  Governor/1(dPm) -> Scope3/1, Mechanical DE/2(dPm)
  PSS1/1(Upss) -> Scope2/1, Excitation System ST1A1/1(Upss)
  Mechanical DE/2(w) -> [f], PSS1/1(w), Governor/1(w)
  "Machine Equations "/2(Igxy1) -> pu->pu/1
  Vgxy/1 -> "Machine Equations "/2(Vgxy)
  "Machine Equations "/4(Vg) -> [Vg], Excitation System ST1A1/3(Vg)
  "Machine Equations "/1(Pe) -> [Pe], Mechanical DE/1(Pe), Scope1/1
  Excitation System ST1A1/1(Ef) -> "Machine Equations "/3(Ef), Scope5/1

== system M10B39_es_V1/Genrators/Generator4 ==
  Vgxy : Inport
  Trip : Inport  Port=2
  Bistable2 : spsBistableLib/Bistable  Qpriority=Set  ic=0  Ts=0
      settings: LibrarySourceBlock=sps_lib/Control/Bistable
  Constant : Constant  Value=[0,0,0,0]
  Excitation System ST1A1 : Subsystem
  Governor : Subsystem
  Ground : Ground
  "Machine Equations " : Subsystem
  Mechanical DE : Subsystem
  Output : Subsystem
  PSS1 : Subsystem
  Scope{,1..3,5} (5 alike) : Scope
  Switch4 : Switch  Criteria=u2 ~= 0  Threshold=0.5  InputSameDT=off
  Terminator : Terminator
  pu->pu : Gain  Gain=SgenB./SgridB
  pu->pu1 : Gain  Gain=SgenB./SgridB
  m : Outport
  Igxy1 : Outport  Port=2
  GBxy : Outport  Port=3
  wires:
  pu->pu1/1 -> [GBxy]
  pu->pu/1 -> [Igxy1]
  "Machine Equations "/3(GBxy) -> Switch4/3
  Constant/1 -> Switch4/1
  Switch4/1 -> pu->pu1/1
  [Trip] -> Switch4/2
  [Trip] -> PSS1/2(Trip)
  [Trip] -> Governor/2(Trip)
  [Trip] -> Mechanical DE/3(Trip)
  [Trip] -> Excitation System ST1A1/2(Trip)
  [Trip] -> "Machine Equations "/4(Trip)
  Bistable2/2 -> Terminator/1
  Trip/1 -> Bistable2/1
  Ground/1 -> Bistable2/2
  Bistable2/1 -> [Trip]
  [Vg] -> Output/6(Vg)
  Output/1(m) -> m/1
  Output/3(GBxy) -> GBxy/1
  Output/2(Igxy1) -> Igxy1/1
  [Igxy1] -> Output/1(Igxy1in)
  [GBxy] -> Output/2(GBxyin)
  [delta] -> Output/3(deltain)
  [f] -> Output/5(fin)
  [Pe] -> Output/4(Pein)
  Mechanical DE/1(delta) -> "Machine Equations "/1(delta), [delta], Scope/1
  Governor/1(dPm) -> Scope3/1, Mechanical DE/2(dPm)
  PSS1/1(Upss) -> Scope2/1, Excitation System ST1A1/1(Upss)
  Mechanical DE/2(w) -> [f], PSS1/1(w), Governor/1(w)
  "Machine Equations "/2(Igxy1) -> pu->pu/1
  Vgxy/1 -> "Machine Equations "/2(Vgxy)
  "Machine Equations "/4(Vg) -> [Vg], Excitation System ST1A1/3(Vg)
  "Machine Equations "/1(Pe) -> [Pe], Mechanical DE/1(Pe), Scope1/1
  Excitation System ST1A1/1(Ef) -> "Machine Equations "/3(Ef), Scope5/1

== system M10B39_es_V1/Genrators/Generator5 ==
  Vgxy : Inport
  Trip : Inport  Port=2
  Bistable2 : spsBistableLib/Bistable  Qpriority=Set  ic=0  Ts=0
      settings: LibrarySourceBlock=sps_lib/Control/Bistable
  Constant : Constant  Value=[0,0,0,0]
  Excitation System ST1A1 : Subsystem
  Governor : Subsystem
  Ground : Ground
  "Machine Equations " : Subsystem
  Mechanical DE : Subsystem
  Output : Subsystem
  PSS1 : Subsystem
  Scope{,1..3,5} (5 alike) : Scope
  Switch4 : Switch  Criteria=u2 ~= 0  Threshold=0.5  InputSameDT=off
  Terminator : Terminator
  pu->pu : Gain  Gain=SgenB./SgridB
  pu->pu1 : Gain  Gain=SgenB./SgridB
  m : Outport
  Igxy1 : Outport  Port=2
  GBxy : Outport  Port=3
  wires:
  pu->pu1/1 -> [GBxy]
  pu->pu/1 -> [Igxy1]
  "Machine Equations "/3(GBxy) -> Switch4/3
  Constant/1 -> Switch4/1
  Switch4/1 -> pu->pu1/1
  [Trip] -> Switch4/2
  [Trip] -> PSS1/2(Trip)
  [Trip] -> Governor/2(Trip)
  [Trip] -> Mechanical DE/3(Trip)
  [Trip] -> Excitation System ST1A1/2(Trip)
  [Trip] -> "Machine Equations "/4(Trip)
  Bistable2/2 -> Terminator/1
  Trip/1 -> Bistable2/1
  Ground/1 -> Bistable2/2
  Bistable2/1 -> [Trip]
  [Vg] -> Output/6(Vg)
  Output/1(m) -> m/1
  Output/3(GBxy) -> GBxy/1
  Output/2(Igxy1) -> Igxy1/1
  [Igxy1] -> Output/1(Igxy1in)
  [GBxy] -> Output/2(GBxyin)
  [delta] -> Output/3(deltain)
  [f] -> Output/5(fin)
  [Pe] -> Output/4(Pein)
  Mechanical DE/1(delta) -> "Machine Equations "/1(delta), [delta], Scope/1
  Governor/1(dPm) -> Scope3/1, Mechanical DE/2(dPm)
  PSS1/1(Upss) -> Scope2/1, Excitation System ST1A1/1(Upss)
  Mechanical DE/2(w) -> [f], PSS1/1(w), Governor/1(w)
  "Machine Equations "/2(Igxy1) -> pu->pu/1
  Vgxy/1 -> "Machine Equations "/2(Vgxy)
  "Machine Equations "/4(Vg) -> [Vg], Excitation System ST1A1/3(Vg)
  "Machine Equations "/1(Pe) -> [Pe], Mechanical DE/1(Pe), Scope1/1
  Excitation System ST1A1/1(Ef) -> "Machine Equations "/3(Ef), Scope5/1

== system M10B39_es_V1/Genrators/ROCOF_ES ==
  Gain14 : Gain  Gain=commun(3,1)
  Gain15 : Gain  Gain=commun(1,2)
  Gain16 : Gain  Gain=commun(2,1)
  Gain18 : Gain  Gain=commun(8,2)
  Gain19 : Gain  Gain=commun(2,2)
  Gain20 : Gain  Gain=commun(5,1)
  Gain21 : Gain  Gain=commun(3,2)
  Gain22 : Gain  Gain=commun(6,1)
  Gain23 : Gain  Gain=commun(4,2)
  Gain24 : Gain  Gain=commun(7,1)
  Gain25 : Gain  Gain=commun(5,2)
  Gain26 : Gain  Gain=commun(8,1)
  Gain27 : Gain  Gain=commun(6,2)
  Gain28 : Gain  Gain=commun(1,1)
  Gain29 : Gain  Gain=commun(7,2)
  Gain9 : Gain  Gain=commun(4,1)
  Mux : Mux  Inputs=2
  Mux15 : Mux
  Mux16 : Mux
  Mux{26..33} (8 alike) : Mux  Inputs=3
  Transport Delay11 : TransportDelay  DelayTime=DataDelay(4,1)
  Transport Delay12 : TransportDelay  DelayTime=DataDelay(5,2)
  Transport Delay13 : TransportDelay  DelayTime=DataDelay(2,1)
  Transport Delay14 : TransportDelay  DelayTime=DataDelay(8,2)
  Transport Delay15 : TransportDelay  DelayTime=DataDelay(1,2)
  Transport Delay18 : TransportDelay  DelayTime=DataDelay(3,1)
  Transport Delay19 : TransportDelay  DelayTime=DataDelay(2,2)
  Transport Delay20 : TransportDelay  DelayTime=DataDelay(5,1)
  Transport Delay21 : TransportDelay  DelayTime=DataDelay(3,2)
  Transport Delay22 : TransportDelay  DelayTime=DataDelay(6,1)
  Transport Delay23 : TransportDelay  DelayTime=DataDelay(4,2)
  Transport Delay24 : TransportDelay  DelayTime=DataDelay(7,1)
  Transport Delay25 : TransportDelay  DelayTime=DataDelay(7,2)
  Transport Delay26 : TransportDelay  DelayTime=DataDelay(8,1)
  Transport Delay27 : TransportDelay  DelayTime=DataDelay(6,2)
  Transport Delay28 : TransportDelay  DelayTime=DataDelay(1,1)
  ROCOF_ES : Outport
  wires:
  Mux27/1 -> Mux15/2  "W_ES2"
  Mux29/1 -> Mux15/4  "W_ES4"
  [DWES1DT] -> Mux26/3  "W1"
  Transport Delay18/1 -> Mux27/1
  Mux16/1 -> Mux/2  "W_ES1"
  Gain22/1 -> Transport Delay22/1
  [DWES2DT] -> Mux27/3  "W2"
  [DWES7DT] -> Gain29/1
  Transport Delay22/1 -> Mux30/1
  Gain26/1 -> Transport Delay26/1
  [DWES8DT] -> Gain18/1  "W4"
  [DWES5DT] -> Mux30/3
  Gain18/1 -> Transport Delay14/1
  [DWES1DT] -> Gain28/1
  [DWES3DT] -> Gain14/1  "W3"
  Mux26/1 -> Mux15/1  "W_ES1"
  Gain19/1 -> Transport Delay19/1
  [DWES8DT] -> Mux33/3
  Gain23/1 -> Transport Delay23/1
  Mux15/1 -> Mux/1  "W_ES1"
  Mux33/1 -> Mux16/4  "W_ES8"
  [DWES1DT] -> Gain15/1  "W1"
  Gain27/1 -> Transport Delay27/1
  [DWES5DT] -> Gain20/1
  Gain9/1 -> Transport Delay11/1
  Gain28/1 -> Transport Delay28/1
  [DWES2DT] -> Gain19/1  "W2"
  Gain29/1 -> Transport Delay25/1
  Transport Delay20/1 -> Mux29/1
  Transport Delay25/1 -> Mux33/2
  [DWES4DT] -> Mux29/3  "W4"
  Transport Delay12/1 -> Mux31/2
  [DWES3DT] -> Mux28/3  "W3"
  Transport Delay28/1 -> Mux33/1
  Transport Delay26/1 -> Mux32/1
  Mux28/1 -> Mux15/3  "W_ES3"
  Transport Delay27/1 -> Mux32/2
  [DWES4DT] -> Gain9/1  "W4"
  [DWES7DT] -> Mux32/3
  [DWES2DT] -> Gain16/1  "W2"
  Mux30/1 -> Mux16/1  "W_ES5"
  [DWES6DT] -> Gain27/1
  Transport Delay13/1 -> Mux26/1
  Transport Delay21/1 -> Mux29/2
  Gain16/1 -> Transport Delay13/1
  Gain14/1 -> Transport Delay18/1
  Transport Delay14/1 -> Mux26/2
  [DWES6DT] -> Gain22/1
  Transport Delay23/1 -> Mux30/2
  Mux/1 -> ROCOF_ES/1
  [DWES3DT] -> Gain21/1  "W3"
  Transport Delay19/1 -> Mux28/2
  [DWES4DT] -> Gain23/1
  Mux31/1 -> Mux16/2  "W_ES6"
  Gain15/1 -> Transport Delay15/1
  Transport Delay15/1 -> Mux27/2
  Gain21/1 -> Transport Delay21/1
  [DWES7DT] -> Gain24/1
  Transport Delay11/1 -> Mux28/1
  Gain20/1 -> Transport Delay20/1
  Gain24/1 -> Transport Delay24/1
  [DWES5DT] -> Gain25/1
  [DWES6DT] -> Mux31/3
  Gain25/1 -> Transport Delay12/1
  Transport Delay24/1 -> Mux31/1
  Mux32/1 -> Mux16/3  "W_ES7"
  [DWES8DT] -> Gain26/1
